simulink model "assigment_3__3_1and3"  (R2022b)
settings: Solver=FixedStepAuto  StartTime=0.0  StopTime=100  FixedStep=0.0001  RelTol=1e-3
settings Model: Creator=iran sistem  LastModifiedBy=iran sistem

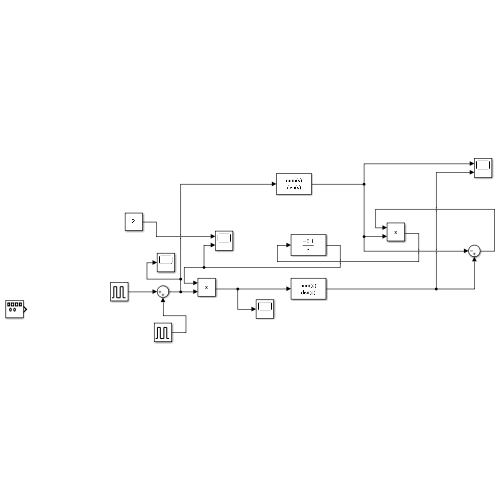
[thumbnail: Simulink's stored preview of the top-level diagram]
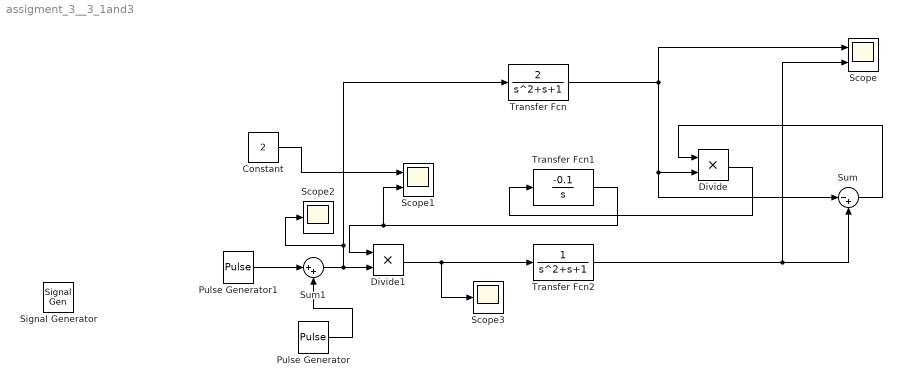
== system assigment_3__3_1and3 ==
  Constant : Constant  Value=2
  Divide : Product  Inputs=**
  Divide1 : Product  Inputs=**
  Pulse Generator : DiscretePulseGenerator  PulseType=Time based  Amplitude=-2.4  Period=20  PulseWidth=50  PhaseDelay=10
  Pulse Generator1 : DiscretePulseGenerator  PulseType=Time based  Amplitude=2.4  Period=20  PulseWidth=50
  Scope : Scope  NumInputPorts=2
  Scope1 : Scope  NumInputPorts=2
  Scope2 : Scope
  Scope3 : Scope
  Signal Generator : SignalGenerator  WaveForm=square  Amplitude=3.5  Units=rad/sec
  Sum : Sum  Inputs=|-+
  Sum1 : Sum  Inputs=|++
  Transfer Fcn : TransferFcn  Numerator=[2]  Denominator=[1 1 1]
  Transfer Fcn1 : TransferFcn  Numerator=[-0.1]  Denominator=[1 0]
  Transfer Fcn2 : TransferFcn  Denominator=[1 1 1]
  wires:
  Divide1/1 -> Scope3/1, Transfer Fcn2/1
  Transfer Fcn1/1 -> Scope1/2, Divide1/1
  Divide/1 -> Transfer Fcn1/1
  Transfer Fcn/1 -> Divide/2, Sum/1, Scope/1
  Transfer Fcn2/1 -> Scope/2, Sum/2
  Sum/1 -> Divide/1
  Constant/1 -> Scope1/1
  Sum1/1 -> Transfer Fcn/1, Scope2/1, Divide1/2
  Pulse Generator1/1 -> Sum1/1
  Pulse Generator/1 -> Sum1/2
